simulink model "bcm_module"  (R2020b)
settings: Solver=VariableStepAuto  StartTime=0.0  StopTime=10  RelTol=1e-3
undefined symbols (not defined in the file): sigbuilder_block
(part 2 of 2)

== system bcm_module/BCM CAR/HVAC/HVAC/Vent ==
  Input : Inport
  Constant1 : Constant  Value=0
  If : If  IfExpression=u1 == 1  ElseIfExpressions=u1 == 2, u1 == 3
  If Action Subsystem : Subsystem  TreatAsAtomicUnit=on
  If Action Subsystem1 : Subsystem  TreatAsAtomicUnit=on
  If Action Subsystem2 : Subsystem  TreatAsAtomicUnit=on
  If Action Subsystem3 : Subsystem  TreatAsAtomicUnit=on
  Signal Builder : Subsystem  Tag=STV Subsys  LoadFcn=sigbuilder_block('load');  StartFcn=sigbuilder_block('start');  StopFcn=sigbuilder_block('stop');  ClipboardFcn=sigbuilder_block('clipboard');  mask(Sigbuilder block){tuvar=[0:10]}
      mask help: Simulink:masks:SigbuilderBlock_MD
      mask init:
      | if ~strcmp(get_param(bdroot(gcbh),'SimulationStatus'),'stopped') tuvar = sigbuilder_block('maskInit'); end
      settings: CopyFcn=sigbuilder_block('copy');  DeleteFcn=sigbuilder_block('delete');  ModelCloseFcn=sigbuilder_block('modelClose');  PreSaveFcn=sigbuilder_block('preSave');  PauseFcn=sigbuilder_block('pause');  ContinueFcn=sigbuilder_block('continue');  NameChangeFcn=sigbuilder_block('namechange');  OpenFcn=sigbuilder_block('open',[437.6 153 550.4 359.25 ]);  CloseFcn=sigbuilder_block('close');
      mask Display: plot(0, 0, 100, 100,[2, 2, 32, 32, 2], [68, 8, 8, 68, 68],[32, 2], [38, 38], [32, 19, 2],[53, 60, 44], [32, 17, 17, 2],[16, 16, 31, 31]);txt = getActiveGroup(gcbh);text(2, 100, txt,'verticalAlignment', 'top');
  Signal Builder1 : Subsystem  Tag=STV Subsys  LoadFcn=sigbuilder_block('load');  StartFcn=sigbuilder_block('start');  StopFcn=sigbuilder_block('stop');  ClipboardFcn=sigbuilder_block('clipboard');  mask(Sigbuilder block){tuvar=[0:10]}
      mask help: Simulink:masks:SigbuilderBlock_MD
      mask init:
      | if ~strcmp(get_param(bdroot(gcbh),'SimulationStatus'),'stopped') tuvar = sigbuilder_block('maskInit'); end
      settings: CopyFcn=sigbuilder_block('copy');  DeleteFcn=sigbuilder_block('delete');  ModelCloseFcn=sigbuilder_block('modelClose');  PreSaveFcn=sigbuilder_block('preSave');  PauseFcn=sigbuilder_block('pause');  ContinueFcn=sigbuilder_block('continue');  NameChangeFcn=sigbuilder_block('namechange');  OpenFcn=sigbuilder_block('open',[437.6 153 550.4 359.25 ]);  CloseFcn=sigbuilder_block('close');
      mask Display: plot(0, 0, 100, 100,[2, 2, 32, 32, 2], [68, 8, 8, 68, 68],[32, 2], [38, 38], [32, 19, 2],[53, 60, 44], [32, 17, 17, 2],[16, 16, 31, 31]);txt = getActiveGroup(gcbh);text(2, 100, txt,'verticalAlignment', 'top');
  Signal Builder2 : Subsystem  Tag=STV Subsys  LoadFcn=sigbuilder_block('load');  StartFcn=sigbuilder_block('start');  StopFcn=sigbuilder_block('stop');  ClipboardFcn=sigbuilder_block('clipboard');  mask(Sigbuilder block){tuvar=[0:10]}
      mask help: Simulink:masks:SigbuilderBlock_MD
      mask init:
      | if ~strcmp(get_param(bdroot(gcbh),'SimulationStatus'),'stopped') tuvar = sigbuilder_block('maskInit'); end
      settings: CopyFcn=sigbuilder_block('copy');  DeleteFcn=sigbuilder_block('delete');  ModelCloseFcn=sigbuilder_block('modelClose');  PreSaveFcn=sigbuilder_block('preSave');  PauseFcn=sigbuilder_block('pause');  ContinueFcn=sigbuilder_block('continue');  NameChangeFcn=sigbuilder_block('namechange');  OpenFcn=sigbuilder_block('open',[437.6 153 550.4 359.25 ]);  CloseFcn=sigbuilder_block('close');
      mask Display: plot(0, 0, 100, 100,[2, 2, 32, 32, 2], [68, 8, 8, 68, 68],[32, 2], [38, 38], [32, 19, 2],[53, 60, 44], [32, 17, 17, 2],[16, 16, 31, 31]);txt = getActiveGroup(gcbh);text(2, 100, txt,'verticalAlignment', 'top');
  Output : Outport
  Output1 : Outport  Port=2
  Output2 : Outport  Port=3
  Output3 : Outport  Port=4
  wires:
  If/4 -> If Action Subsystem3/Action
  If/2 -> If Action Subsystem1/Action
  Signal Builder2/1(Signal 1) -> If Action Subsystem2/1(In1)
  Constant1/1 -> If Action Subsystem3/1(In1)
  Input/1 -> If/1
  Signal Builder/1(Signal 2) -> If Action Subsystem/1(In1)
  If/3 -> If Action Subsystem2/Action
  If/1 -> If Action Subsystem/Action
  If Action Subsystem1/1(Out1) -> Output1/1
  Signal Builder1/1(Signal 2) -> If Action Subsystem1/1(In1)
  If Action Subsystem/1(Output) -> Output/1
  If Action Subsystem2/1(Output2) -> Output2/1
  If Action Subsystem3/1(Output3) -> Output3/1

== system bcm_module/BCM CAR/Seat_subsystem/Front_Left/Horizontal_Direction ==
  In1 : Inport
  Add : Sum
  Add1 : Sum
  Cond_check : Constant
  Cond_check1 : Constant  Value=-1
  Cond_check3 : Constant  Value=0
  If Action Subsystem : Subsystem  TreatAsAtomicUnit=on
  If Action Subsystem1 : Subsystem  TreatAsAtomicUnit=on
  If Action Subsystem2 : Subsystem  TreatAsAtomicUnit=on
  Unit Delay : UnitDelay  SampleTime=-1  HasFrameUpgradeWarning=on
  Unit Delay1 : UnitDelay  SampleTime=-1  HasFrameUpgradeWarning=on
  check_user_input : If  IfExpression=u1 == 1  ElseIfExpressions=u1 == -1
  mov_for : Outport
  mov_back : Outport  Port=2
  stay : Outport  Port=3
  wires:
  In1/1 -> check_user_input/1  "User_input"
  check_user_input/1 -> If Action Subsystem/Action
  Cond_check/1 -> If Action Subsystem/1(In1)
  Cond_check1/1 -> If Action Subsystem1/1(In1)
  check_user_input/3 -> If Action Subsystem2/Action
  check_user_input/2 -> If Action Subsystem1/Action
  Cond_check3/1 -> If Action Subsystem2/1(In1)
  If Action Subsystem2/1(Out1) -> stay/1
  Unit Delay/1 -> Add/2
  Add/1 -> mov_for/1, Unit Delay/1
  If Action Subsystem/1(Out1) -> Add/1
  Unit Delay1/1 -> Add1/2
  Add1/1 -> mov_back/1, Unit Delay1/1
  If Action Subsystem1/1(Out1) -> Add1/1

== system bcm_module/BCM CAR/Seat_subsystem/Front_Left/Vertical_Direction ==
  user_input : Inport
  Add : Sum
  Add1 : Sum
  Cond_check : Constant
  Cond_check1 : Constant  Value=-1
  Cond_check3 : Constant  Value=0
  If Action Subsystem : Subsystem  TreatAsAtomicUnit=on
  If Action Subsystem1 : Subsystem  TreatAsAtomicUnit=on
  If Action Subsystem2 : Subsystem  TreatAsAtomicUnit=on
  Unit Delay : UnitDelay  SampleTime=-1  HasFrameUpgradeWarning=on
  Unit Delay1 : UnitDelay  SampleTime=-1  HasFrameUpgradeWarning=on
  check_user_input : If  IfExpression=u1 == 1  ElseIfExpressions=u1 == -1
  mov_up : Outport
  mov_down : Outport  Port=2
  stay : Outport  Port=3
  wires:
  If Action Subsystem2/1(Out1) -> stay/1
  check_user_input/2 -> If Action Subsystem1/Action
  Cond_check3/1 -> If Action Subsystem2/1(In1)
  Cond_check/1 -> If Action Subsystem/1(In1)
  check_user_input/3 -> If Action Subsystem2/Action
  Cond_check1/1 -> If Action Subsystem1/1(In1)
  check_user_input/1 -> If Action Subsystem/Action
  user_input/1 -> check_user_input/1
  Unit Delay/1 -> Add/2
  Add/1 -> mov_down/1, Unit Delay/1
  If Action Subsystem1/1(Out1) -> Add/1
  Unit Delay1/1 -> Add1/2
  Add1/1 -> mov_up/1, Unit Delay1/1
  If Action Subsystem/1(Out1) -> Add1/1

== system bcm_module/BCM CAR/Seat_subsystem/Front_Right/Horizontal_Direction ==
  In1 : Inport
  Add : Sum
  Add1 : Sum
  Cond_check : Constant
  Cond_check1 : Constant  Value=-1
  Cond_check3 : Constant  Value=0
  If Action Subsystem : Subsystem  TreatAsAtomicUnit=on
  If Action Subsystem1 : Subsystem  TreatAsAtomicUnit=on
  If Action Subsystem2 : Subsystem  TreatAsAtomicUnit=on
  Unit Delay : UnitDelay  SampleTime=-1  HasFrameUpgradeWarning=on
  Unit Delay1 : UnitDelay  SampleTime=-1  HasFrameUpgradeWarning=on
  check_user_input : If  IfExpression=u1 == 1  ElseIfExpressions=u1 == -1
  mov_for : Outport
  mov_back : Outport  Port=2
  stay : Outport  Port=3
  wires:
  In1/1 -> check_user_input/1  "User_input"
  check_user_input/1 -> If Action Subsystem/Action
  Cond_check/1 -> If Action Subsystem/1(In1)
  Cond_check1/1 -> If Action Subsystem1/1(In1)
  check_user_input/3 -> If Action Subsystem2/Action
  check_user_input/2 -> If Action Subsystem1/Action
  Cond_check3/1 -> If Action Subsystem2/1(In1)
  If Action Subsystem2/1(Out1) -> stay/1
  Unit Delay/1 -> Add/2
  Add/1 -> mov_for/1, Unit Delay/1
  If Action Subsystem/1(Out1) -> Add/1
  Unit Delay1/1 -> Add1/2
  Add1/1 -> mov_back/1, Unit Delay1/1
  If Action Subsystem1/1(Out1) -> Add1/1

== system bcm_module/BCM CAR/Seat_subsystem/Front_Right/Vertical_Direction ==
  user_input : Inport
  Add : Sum
  Add1 : Sum
  Cond_check : Constant
  Cond_check1 : Constant  Value=-1
  Cond_check3 : Constant  Value=0
  If Action Subsystem : Subsystem  TreatAsAtomicUnit=on
  If Action Subsystem1 : Subsystem  TreatAsAtomicUnit=on
  If Action Subsystem2 : Subsystem  TreatAsAtomicUnit=on
  Unit Delay : UnitDelay  SampleTime=-1  HasFrameUpgradeWarning=on
  Unit Delay1 : UnitDelay  SampleTime=-1  HasFrameUpgradeWarning=on
  check_user_input : If  IfExpression=u1 == 1  ElseIfExpressions=u1 == -1
  mov_up : Outport
  mov_back : Outport  Port=2
  stay : Outport  Port=3
  wires:
  If Action Subsystem2/1(Out1) -> stay/1
  check_user_input/2 -> If Action Subsystem1/Action
  Cond_check3/1 -> If Action Subsystem2/1(In1)
  Cond_check/1 -> If Action Subsystem/1(In1)
  check_user_input/3 -> If Action Subsystem2/Action
  Cond_check1/1 -> If Action Subsystem1/1(In1)
  check_user_input/1 -> If Action Subsystem/Action
  user_input/1 -> check_user_input/1
  Unit Delay/1 -> Add/2
  Add/1 -> mov_back/1, Unit Delay/1
  If Action Subsystem1/1(Out1) -> Add/1
  Unit Delay1/1 -> Add1/2
  Add1/1 -> mov_up/1, Unit Delay1/1
  If Action Subsystem/1(Out1) -> Add1/1

== system bcm_module/BCM CAR/Wiper Subsystem/First wiper/If Action Subsystem ==
  In1 : Inport
  Action Port : ActionPort  ActionPortLabel=if(u1<=20)
  Out1 : Outport
  wires:
  In1/1 -> Out1/1

== system bcm_module/BCM CAR/Wiper Subsystem/First wiper/If Action Subsystem1 ==
  In1 : Inport
  Action Port : ActionPort  ActionPortLabel=elseif(u1<=40)
  Out1 : Outport
  wires:
  In1/1 -> Out1/1

== system bcm_module/BCM CAR/Wiper Subsystem/First wiper/If Action Subsystem2 ==
  In1 : Inport
  Action Port : ActionPort  ActionPortLabel=elseif(u1<=60)
  Out1 : Outport
  wires:
  In1/1 -> Out1/1

== system bcm_module/BCM CAR/Wiper Subsystem/First wiper/If Action Subsystem3 ==
  In1 : Inport
  Action Port : ActionPort  ActionPortLabel=else
  Out1 : Outport
  wires:
  In1/1 -> Out1/1

== system bcm_module/BCM CAR/Wiper Subsystem/Secod wiper/If Action Subsystem ==
  In1 : Inport
  Action Port : ActionPort  ActionPortLabel=if(u1<=20)
  Out1 : Outport
  wires:
  In1/1 -> Out1/1

== system bcm_module/BCM CAR/Wiper Subsystem/Secod wiper/If Action Subsystem1 ==
  In1 : Inport
  Action Port : ActionPort  ActionPortLabel=elseif(u1<=40)
  Out1 : Outport
  wires:
  In1/1 -> Out1/1

== system bcm_module/BCM CAR/Wiper Subsystem/Secod wiper/If Action Subsystem2 ==
  In1 : Inport
  Action Port : ActionPort  ActionPortLabel=elseif(u1<=60)
  Out1 : Outport
  wires:
  In1/1 -> Out1/1

== system bcm_module/BCM CAR/Wiper Subsystem/Secod wiper/If Action Subsystem3 ==
  In1 : Inport
  Action Port : ActionPort  ActionPortLabel=else
  Out1 : Outport
  wires:
  In1/1 -> Out1/1

== system bcm_module/BCM CAR/mirror/left_mirror/If Action Subsystem ==
  In1 : Inport
  Action Port : ActionPort  ActionPortLabel=if(u1 == 1)
  Out1 : Outport
  wires:
  In1/1 -> Out1/1

== system bcm_module/BCM CAR/mirror/left_mirror/If Action Subsystem1 ==
  In1 : Inport
  Action Port : ActionPort  ActionPortLabel=elseif( u1 == 2)
  Out1 : Outport
  wires:
  In1/1 -> Out1/1

== system bcm_module/BCM CAR/mirror/left_mirror/If Action Subsystem2 ==
  In1 : Inport
  Action Port : ActionPort  ActionPortLabel=elseif(u1 == -1 )
  Out1 : Outport
  wires:
  In1/1 -> Out1/1

== system bcm_module/BCM CAR/mirror/left_mirror/If Action Subsystem3 ==
  In1 : Inport
  Action Port : ActionPort  ActionPortLabel=else
  Out1 : Outport
  wires:
  In1/1 -> Out1/1

== system bcm_module/BCM CAR/mirror/right_mirror/If Action Subsystem ==
  In1 : Inport
  Action Port : ActionPort  ActionPortLabel=if(u1 == 1)
  Out1 : Outport
  wires:
  In1/1 -> Out1/1

== system bcm_module/BCM CAR/mirror/right_mirror/If Action Subsystem1 ==
  In1 : Inport
  Action Port : ActionPort  ActionPortLabel=elseif( u1 == 2)
  Out1 : Outport
  wires:
  In1/1 -> Out1/1

== system bcm_module/BCM CAR/mirror/right_mirror/If Action Subsystem2 ==
  In1 : Inport
  Action Port : ActionPort  ActionPortLabel=elseif(u1 == -1 )
  Out1 : Outport
  wires:
  In1/1 -> Out1/1

== system bcm_module/BCM CAR/mirror/right_mirror/If Action Subsystem3 ==
  In1 : Inport
  Action Port : ActionPort  ActionPortLabel=else
  Out1 : Outport
  wires:
  In1/1 -> Out1/1

== system bcm_module/BCM CAR/power_window/Back_left_passenger/Do Nothing ==
  In1 : Inport
  Action Port : ActionPort  ActionPortLabel=default:
  Out1 : Outport
  wires:
  In1/1 -> Out1/1

== system bcm_module/BCM CAR/power_window/Back_left_passenger/Long Down ==
  In1 : Inport
  Action Port : ActionPort  ActionPortLabel=case [ 4 ]:
  Out1 : Outport
  wires:
  In1/1 -> Out1/1

== system bcm_module/BCM CAR/power_window/Back_left_passenger/Long Up ==
  In1 : Inport
  Action Port : ActionPort  ActionPortLabel=case [ 1 ]:
  Out1 : Outport
  wires:
  In1/1 -> Out1/1

== system bcm_module/BCM CAR/power_window/Back_left_passenger/Short Down ==
  In1 : Inport
  Action Port : ActionPort  ActionPortLabel=case [ 3 ]:
  Out1 : Outport
  wires:
  In1/1 -> Out1/1

== system bcm_module/BCM CAR/power_window/Back_left_passenger/Short Up ==
  In1 : Inport
  Action Port : ActionPort  ActionPortLabel=case [ 2 ]:
  Out1 : Outport
  wires:
  In1/1 -> Out1/1

== system bcm_module/BCM CAR/power_window/Back_right_passenger/Do Nothing ==
  In1 : Inport
  Action Port : ActionPort  ActionPortLabel=default:
  Out1 : Outport
  wires:
  In1/1 -> Out1/1

== system bcm_module/BCM CAR/power_window/Back_right_passenger/Long Down ==
  In1 : Inport
  Action Port : ActionPort  ActionPortLabel=case [ 4 ]:
  Out1 : Outport
  wires:
  In1/1 -> Out1/1

== system bcm_module/BCM CAR/power_window/Back_right_passenger/Long Up ==
  In1 : Inport
  Action Port : ActionPort  ActionPortLabel=case [ 1 ]:
  Out1 : Outport
  wires:
  In1/1 -> Out1/1

== system bcm_module/BCM CAR/power_window/Back_right_passenger/Short Down ==
  In1 : Inport
  Action Port : ActionPort  ActionPortLabel=case [ 3 ]:
  Out1 : Outport
  wires:
  In1/1 -> Out1/1

== system bcm_module/BCM CAR/power_window/Back_right_passenger/Short Up ==
  In1 : Inport
  Action Port : ActionPort  ActionPortLabel=case [ 2 ]:
  Out1 : Outport
  wires:
  In1/1 -> Out1/1

== system bcm_module/BCM CAR/power_window/driver_button/Do_Nothing ==
  In1 : Inport
  Action Port : ActionPort  ActionPortLabel=default:
  Out1 : Outport
  wires:
  In1/1 -> Out1/1

== system bcm_module/BCM CAR/power_window/driver_button/Long_Down ==
  In1 : Inport
  Action Port : ActionPort  ActionPortLabel=case [ 4 ]:
  Out1 : Outport
  wires:
  In1/1 -> Out1/1

== system bcm_module/BCM CAR/power_window/driver_button/Long_Up ==
  In1 : Inport
  Action Port : ActionPort  ActionPortLabel=case [ 1 ]:
  Out1 : Outport
  wires:
  In1/1 -> Out1/1

== system bcm_module/BCM CAR/power_window/driver_button/Short_Down ==
  In1 : Inport
  Action Port : ActionPort  ActionPortLabel=case [ 3 ]:
  Out1 : Outport
  wires:
  In1/1 -> Out1/1

== system bcm_module/BCM CAR/power_window/driver_button/Short_Up ==
  In1 : Inport
  Action Port : ActionPort  ActionPortLabel=case [ 2 ]:
  Out1 : Outport
  wires:
  In1/1 -> Out1/1

== system bcm_module/BCM CAR/power_window/front_passenger/Do Nothing ==
  In1 : Inport
  Action Port : ActionPort  ActionPortLabel=default:
  Out1 : Outport
  wires:
  In1/1 -> Out1/1

== system bcm_module/BCM CAR/power_window/front_passenger/Long Down ==
  In1 : Inport
  Action Port : ActionPort  ActionPortLabel=case [ 4 ]:
  Out1 : Outport
  wires:
  In1/1 -> Out1/1

== system bcm_module/BCM CAR/power_window/front_passenger/Long Up ==
  In1 : Inport
  Action Port : ActionPort  ActionPortLabel=case [ 1 ]:
  Out1 : Outport
  wires:
  In1/1 -> Out1/1

== system bcm_module/BCM CAR/power_window/front_passenger/Short Down ==
  In1 : Inport
  Action Port : ActionPort  ActionPortLabel=case [ 3 ]:
  Out1 : Outport
  wires:
  In1/1 -> Out1/1

== system bcm_module/BCM CAR/power_window/front_passenger/Short Up ==
  In1 : Inport
  Action Port : ActionPort  ActionPortLabel=case [ 2 ]:
  Out1 : Outport
  wires:
  In1/1 -> Out1/1

== system bcm_module/BCM CAR/HVAC/HVAC/Cooler/If Action Subsystem ==
  In1 : Inport
  Action Port : ActionPort  ActionPortLabel=if(u1 == 1)
  Out1 : Outport
  wires:
  In1/1 -> Out1/1

== system bcm_module/BCM CAR/HVAC/HVAC/Cooler/If Action Subsystem1 ==
  In1 : Inport
  Action Port : ActionPort  ActionPortLabel=elseif(u1 == 2)
  Output1 : Outport
  wires:
  In1/1 -> Output1/1

== system bcm_module/BCM CAR/HVAC/HVAC/Cooler/If Action Subsystem2 ==
  In1 : Inport
  Action Port : ActionPort  ActionPortLabel=elseif( u1 == 3)
  Out1 : Outport
  wires:
  In1/1 -> Out1/1

== system bcm_module/BCM CAR/HVAC/HVAC/Cooler/If Action Subsystem3 ==
  In1 : Inport
  Action Port : ActionPort  ActionPortLabel=else
  Out1 : Outport
  wires:
  In1/1 -> Out1/1

== system bcm_module/BCM CAR/HVAC/HVAC/Heater/If Action Subsystem ==
  In1 : Inport
  Action Port : ActionPort  ActionPortLabel=if(u1 == 1)
  Output : Outport
  wires:
  In1/1 -> Output/1

== system bcm_module/BCM CAR/HVAC/HVAC/Heater/If Action Subsystem1 ==
  In1 : Inport
  Action Port : ActionPort  ActionPortLabel=elseif(u1 == 2)
  Out1 : Outport
  wires:
  In1/1 -> Out1/1

== system bcm_module/BCM CAR/HVAC/HVAC/Heater/If Action Subsystem2 ==
  In1 : Inport
  Action Port : ActionPort  ActionPortLabel=elseif( u1 == 3)
  Out1 : Outport
  wires:
  In1/1 -> Out1/1

== system bcm_module/BCM CAR/HVAC/HVAC/Heater/If Action Subsystem3 ==
  In1 : Inport
  Action Port : ActionPort  ActionPortLabel=else
  Out1 : Outport
  wires:
  In1/1 -> Out1/1

== system bcm_module/BCM CAR/HVAC/HVAC/Heater/Signal Builder1 ==
  Demux : Demux  Tag=STV Demux  Outputs=1
      settings: DisplayOption=none
  FromWs : FromWorkspace  Tag=STV FromWs  VariableName=tuvar
      SigBuilderData=|
      | common.afterFinalStr = 'Extrapolate'
      | common.sampleTime = 0
      | dataSet.timeRange = [0 10]
      | dataSet.name = 'Group 1'
      | sbobj.Groups.Name = 'Group 1'
      | sbobj.Groups.Signals.Name = 'Signal 2'
      | sbobj.Groups.Signals.XData = [0 0.5 0.5 1 1 1.5 1.5 2 2 2.5 2.5 3 3 3.5 3.5 4 4 4.5 4.5 5 5 5.5 5.5 6 6 6.5 6.5 7 7 7.5 7.5 8 8 8.5 8.5 9 9 9.5 9.5 10]
      | sbobj.Groups.Signals.YData = [2 2 0 0 2 2 0 0 2 2 0 0 2 2 0 0 2 2 0 0 2 2 0 0 2 2 0 0 2 2 0 0 2 2 0 0 2 2 0 0]
  Signal 2 : Outport  Tag=STV Outport
  wires:
  FromWs/1 -> Demux/1
  Demux/1 -> Signal 2/1

== system bcm_module/BCM CAR/HVAC/HVAC/Heater/Signal Builder2 ==
  Demux : Demux  Tag=STV Demux  Outputs=1
      settings: DisplayOption=none
  FromWs : FromWorkspace  Tag=STV FromWs  VariableName=tuvar
      SigBuilderData=|
      | common.afterFinalStr = 'Extrapolate'
      | common.sampleTime = 0
      | dataSet.timeRange = [0 10]
      | dataSet.name = 'Group 1'
      | sbobj.Groups.Name = 'Group 1'
      | sbobj.Groups.Signals.Name = 'Signal 1'
      | sbobj.Groups.Signals.XData = [0 0.75 0.75 1 1 1.75 1.75 2 2 2.75 2.75 3 3 3.75 3.75 4 4 4.75 4.75 5 5 5.75 5.75 6 6 6.75 6.75 7 7 7.75 7.75 8 8 8.75 8.75 9 9 9.75 9.75 10]
      | sbobj.Groups.Signals.YData = [2 2 0 0 2 2 0 0 2 2 0 0 2 2 0 0 2 2 0 0 2 2 0 0 2 2 0 0 2 2 0 0 2 2 0 0 2 2 0 0]
  Signal 1 : Outport  Tag=STV Outport
  wires:
  FromWs/1 -> Demux/1
  Demux/1 -> Signal 1/1

== system bcm_module/BCM CAR/HVAC/HVAC/Vent/If Action Subsystem ==
  In1 : Inport
  Action Port : ActionPort  ActionPortLabel=if(u1 == 1)
  Output : Outport
  wires:
  In1/1 -> Output/1

== system bcm_module/BCM CAR/HVAC/HVAC/Vent/If Action Subsystem1 ==
  In1 : Inport
  Action Port : ActionPort  ActionPortLabel=elseif(u1 == 2)
  Out1 : Outport
  wires:
  In1/1 -> Out1/1

== system bcm_module/BCM CAR/HVAC/HVAC/Vent/If Action Subsystem2 ==
  In1 : Inport
  Action Port : ActionPort  ActionPortLabel=elseif( u1 == 3)
  Output2 : Outport
  wires:
  In1/1 -> Output2/1

== system bcm_module/BCM CAR/HVAC/HVAC/Vent/If Action Subsystem3 ==
  In1 : Inport
  Action Port : ActionPort  ActionPortLabel=else
  Output3 : Outport
  wires:
  In1/1 -> Output3/1

== system bcm_module/BCM CAR/HVAC/HVAC/Vent/Signal Builder ==
  Demux : Demux  Tag=STV Demux  Outputs=1
      settings: DisplayOption=none
  FromWs : FromWorkspace  Tag=STV FromWs  VariableName=tuvar
      SigBuilderData=|
      | common.afterFinalStr = 'Extrapolate'
      | common.sampleTime = 0
      | dataSet.timeRange = [0 10]
      | dataSet.name = 'Group 1'
      | sbobj.Groups.Name = 'Group 1'
      | sbobj.Groups.Signals.Name = 'Signal 2'
      | sbobj.Groups.Signals.XData = [0 0.25 0.25 1 1 1.25 1.25 2 2 2.25 2.25 3 3 3.25 3.25 4 4 4.25 4.25 5 5 5.25 5.25 6 6 6.25 6.25 7 7 7.25 7.25 8 8 8.25 8.25 9 9 9.25 9.25 10]
      | sbobj.Groups.Signals.YData = [2 2 0 0 2 2 0 0 2 2 0 0 2 2 0 0 2 2 0 0 2 2 0 0 2 2 0 0 2 2 0 0 2 2 0 0 2 2 0 0]
  Signal 2 : Outport  Tag=STV Outport
  wires:
  FromWs/1 -> Demux/1
  Demux/1 -> Signal 2/1

== system bcm_module/BCM CAR/HVAC/HVAC/Vent/Signal Builder1 ==
  Demux : Demux  Tag=STV Demux  Outputs=1
      settings: DisplayOption=none
  FromWs : FromWorkspace  Tag=STV FromWs  VariableName=tuvar
      SigBuilderData=|
      | common.afterFinalStr = 'Extrapolate'
      | common.sampleTime = 0
      | dataSet.timeRange = [0 10]
      | dataSet.name = 'Group 1'
      | sbobj.Groups.Name = 'Group 1'
      | sbobj.Groups.Signals.Name = 'Signal 2'
      | sbobj.Groups.Signals.XData = [0 0.5 0.5 1 1 1.5 1.5 2 2 2.5 2.5 3 3 3.5 3.5 4 4 4.5 4.5 5 5 5.5 5.5 6 6 6.5 6.5 7 7 7.5 7.5 8 8 8.5 8.5 9 9 9.5 9.5 10]
      | sbobj.Groups.Signals.YData = [2 2 0 0 2 2 0 0 2 2 0 0 2 2 0 0 2 2 0 0 2 2 0 0 2 2 0 0 2 2 0 0 2 2 0 0 2 2 0 0]
  Signal 2 : Outport  Tag=STV Outport
  wires:
  FromWs/1 -> Demux/1
  Demux/1 -> Signal 2/1

== system bcm_module/BCM CAR/HVAC/HVAC/Vent/Signal Builder2 ==
  Demux : Demux  Tag=STV Demux  Outputs=1
      settings: DisplayOption=none
  FromWs : FromWorkspace  Tag=STV FromWs  VariableName=tuvar
      SigBuilderData=|
      | common.afterFinalStr = 'Extrapolate'
      | common.sampleTime = 0
      | dataSet.timeRange = [0 10]
      | dataSet.name = 'Group 1'
      | sbobj.Groups.Name = 'Group 1'
      | sbobj.Groups.Signals.Name = 'Signal 1'
      | sbobj.Groups.Signals.XData = [0 0.75 0.75 1 1 1.75 1.75 2 2 2.75 2.75 3 3 3.75 3.75 4 4 4.75 4.75 5 5 5.75 5.75 6 6 6.75 6.75 7 7 7.75 7.75 8 8 8.75 8.75 9 9 9.75 9.75 10]
      | sbobj.Groups.Signals.YData = [2 2 0 0 2 2 0 0 2 2 0 0 2 2 0 0 2 2 0 0 2 2 0 0 2 2 0 0 2 2 0 0 2 2 0 0 2 2 0 0]
  Signal 1 : Outport  Tag=STV Outport
  wires:
  FromWs/1 -> Demux/1
  Demux/1 -> Signal 1/1

== system bcm_module/BCM CAR/Seat_subsystem/Front_Left/Horizontal_Direction/If Action Subsystem ==
  In1 : Inport
  Action Port : ActionPort  ActionPortLabel=if(u1 == 1)
  Out1 : Outport
  wires:
  In1/1 -> Out1/1

== system bcm_module/BCM CAR/Seat_subsystem/Front_Left/Horizontal_Direction/If Action Subsystem1 ==
  In1 : Inport
  Action Port : ActionPort  ActionPortLabel=elseif(u1 == -1)
  Out1 : Outport
  wires:
  In1/1 -> Out1/1

== system bcm_module/BCM CAR/Seat_subsystem/Front_Left/Horizontal_Direction/If Action Subsystem2 ==
  In1 : Inport
  Action Port : ActionPort  ActionPortLabel=else
  Out1 : Outport
  wires:
  In1/1 -> Out1/1

== system bcm_module/BCM CAR/Seat_subsystem/Front_Left/Vertical_Direction/If Action Subsystem ==
  In1 : Inport
  Action Port : ActionPort  ActionPortLabel=if(u1 == 1)
  Out1 : Outport
  wires:
  In1/1 -> Out1/1

== system bcm_module/BCM CAR/Seat_subsystem/Front_Left/Vertical_Direction/If Action Subsystem1 ==
  In1 : Inport
  Action Port : ActionPort  ActionPortLabel=elseif(u1 == -1)
  Out1 : Outport
  wires:
  In1/1 -> Out1/1

== system bcm_module/BCM CAR/Seat_subsystem/Front_Left/Vertical_Direction/If Action Subsystem2 ==
  In1 : Inport
  Action Port : ActionPort  ActionPortLabel=else
  Out1 : Outport
  wires:
  In1/1 -> Out1/1

== system bcm_module/BCM CAR/Seat_subsystem/Front_Right/Horizontal_Direction/If Action Subsystem ==
  In1 : Inport
  Action Port : ActionPort  ActionPortLabel=if(u1 == 1)
  Out1 : Outport
  wires:
  In1/1 -> Out1/1

== system bcm_module/BCM CAR/Seat_subsystem/Front_Right/Horizontal_Direction/If Action Subsystem1 ==
  In1 : Inport
  Action Port : ActionPort  ActionPortLabel=elseif(u1 == -1)
  Out1 : Outport
  wires:
  In1/1 -> Out1/1

== system bcm_module/BCM CAR/Seat_subsystem/Front_Right/Horizontal_Direction/If Action Subsystem2 ==
  In1 : Inport
  Action Port : ActionPort  ActionPortLabel=else
  Out1 : Outport
  wires:
  In1/1 -> Out1/1

== system bcm_module/BCM CAR/Seat_subsystem/Front_Right/Vertical_Direction/If Action Subsystem ==
  In1 : Inport
  Action Port : ActionPort  ActionPortLabel=if(u1 == 1)
  Out1 : Outport
  wires:
  In1/1 -> Out1/1

== system bcm_module/BCM CAR/Seat_subsystem/Front_Right/Vertical_Direction/If Action Subsystem1 ==
  In1 : Inport
  Action Port : ActionPort  ActionPortLabel=elseif(u1 == -1)
  Out1 : Outport
  wires:
  In1/1 -> Out1/1

== system bcm_module/BCM CAR/Seat_subsystem/Front_Right/Vertical_Direction/If Action Subsystem2 ==
  In1 : Inport
  Action Port : ActionPort  ActionPortLabel=else
  Out1 : Outport
  wires:
  In1/1 -> Out1/1
